simulink model "pitch_attitude_SP"  (R2017a)
settings: Solver=ode4  StartTime=0.0  StopTime=SimTime  FixedStep=stepSize  RelTol=1e-3
values from neighbouring files (symbols this model uses):
  K_theta_damping = 20    [AE168_project.m]
  K_thetadot = 6.5    [AE168_project.m]
  tau = 0.1    [AE168_project.m]
undefined symbols (not defined in the file or in its folder): q_den, q_num
libraries: simulink_extras x2
settings Model: Creator=Jeremiah  LastModifiedBy=Jeremiah
settings SolverCC: InitialStep=stepSize

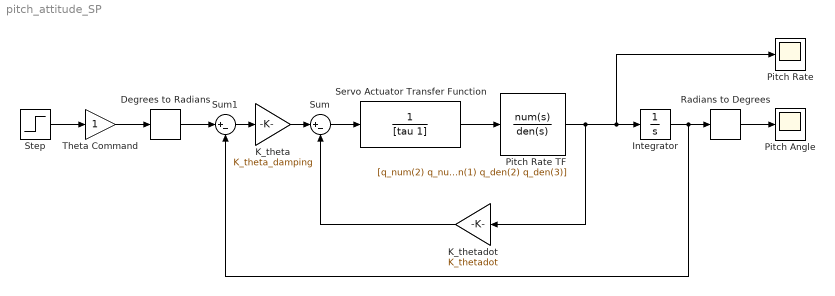
== system pitch_attitude_SP ==
  Degrees to Radians : simulink_extras/Transformations/Degrees to Radians
  Integrator : Integrator
  K_theta : Gain  Gain=K_theta_damping
  K_thetadot : Gain  Gain=K_thetadot
  Pitch Angle : Scope
  Pitch Rate : Scope
  Pitch Rate TF : TransferFcn  Numerator=[q_num(2) q_num(3)]  Denominator=[q_den(1) q_den(2) q_den(3)]  ContinuousStateAttributes='pitch_rate'
  Radians to Degrees : simulink_extras/Transformations/Radians to Degrees
  Servo Actuator Transfer Function : TransferFcn  Denominator=[tau 1]  ContinuousStateAttributes='pitch_attitude'
  Step : Step  Time=0  SampleTime=0.1
  Sum : Sum  Inputs=|+-
  Sum1 : Sum  Inputs=|+-
  Theta Command : Gain
  wires:
  Theta Command/1 -> Degrees to Radians/1
  Radians to Degrees/1 -> Pitch Angle/1
  Step/1 -> Theta Command/1
  Pitch Rate TF/1 -> Pitch Rate/1, Integrator/1, K_thetadot/1
  Integrator/1 -> Sum1/2, Radians to Degrees/1
  Servo Actuator Transfer Function/1 -> Pitch Rate TF/1
  K_thetadot/1 -> Sum/2
  Sum/1 -> Servo Actuator Transfer Function/1
  K_theta/1 -> Sum/1
  Degrees to Radians/1 -> Sum1/1
  Sum1/1 -> K_theta/1
